simulink model "afe_abc_inv_pmsm"  (R2024b)
settings: Solver=ode1be  StartTime=0.0  StopTime=simlength  FixedStep=tc  MaxStep=tc
undefined symbols (not defined in the file): Adrso, Amplitude_U, Amplitude_V, Amplitude_W, Aresd, b, Bresd, Cresd, Crso, CTRPIFF_CLIP_RELEASE, dead_time_AFE, dead_time_INV, deepNEGeta, deepNEGxi, deepPOSxi, emf_fb_p, emf_fb_p_ccaller_1, emf_fb_p_ccaller_2, emf_p, emf_p_ccaller_1, emf_p_ccaller_2, end_time_LVRT, fPWM_AFE, fPWM_INV, g0_161Hz, g0_500Hz, g1_161Hz, g1_500Hz, i_grid_neg_eta_lim, i_grid_neg_eta_red_lim, i_grid_neg_xi_lim, i_grid_neg_xi_red_lim, i_grid_pos_eta_lim, i_grid_pos_eta_red_lim, ibez, id_lim, ieta_neg_ref_lim, ieta_pos_ref_lim, Igrid_phase_normalization_factor, iq_lim, ixi_pos_ref_lim, Jm, k_frt_ref, kg, ki_afe, ki_i, ki_rc_neg_grid, ki_rc_pos_grid, ki_vs, ki_w, kp_afe, kp_i, kp_rc_neg_grid, kp_rc_pos_grid, kp_vs, kp_w, kw, l1, l2, Ld_norm ... (+45)
libraries: fl_lib x115, nesl_utility x75, cstblocks x14, simulink x13, single_phase_transformer_lib x3, threephase_inductor_lib x2, flexshaft_lib x1, pmsm_uvw_with_harmonics_lib x1
(part 8 of 10)

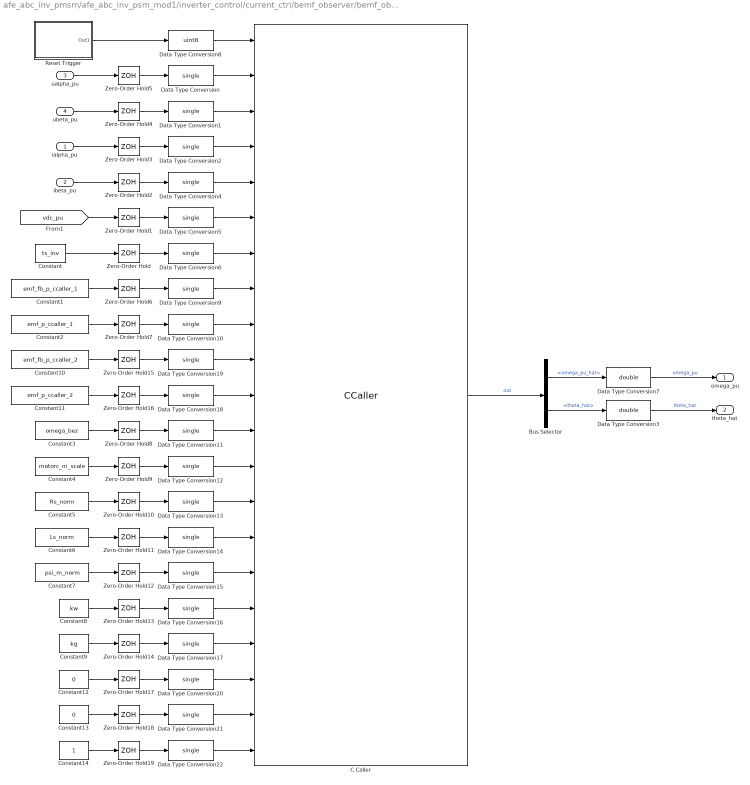
== system afe_abc_inv_pmsm/afe_abc_inv_psm_mod1/inverter_control/current_ctrl/bemf_observer/bemf_observer_ccaller ==
  ialpha_pu : Inport
  ibeta_pu : Inport  Port=2
  ualpha_pu : Inport  Port=3
  ubeta_pu : Inport  Port=4
  Bus Selector : BusSelector  OutputSignals=omega_pu_hat,theta_hat
  C Caller : CCaller  FunctionName=bemf_obsv_process_simulink  PortSpecificationStruct="%)30     .    N\"8   8    (     @         %    \"    !8    !     0         %  0 \"0    $    _    07)G3F%M90  4&]R=$YA;64 4V-O<&4     26YD97@     5'EP90      4VEZ90      27-';&]B86P   X    P    !@    @    $          4    (     0    ,    !         !   P!O=70 #@   #     &    \"     0         !0    @    !     P    $         $  # &]U=  .    .     8    (    !          %    \"     $    &     0         0  ...(+12985 chars)"  SampleTime=ts_inv
  Constant : Constant  Value=ts_inv
  Constant1 : Constant  Value=emf_fb_p_ccaller_1
  Constant10 : Constant  Value=emf_fb_p_ccaller_2
  Constant11 : Constant  Value=emf_p_ccaller_2
  Constant12 : Constant  Value=0
  Constant13 : Constant  Value=0
  Constant14 : Constant
  Constant2 : Constant  Value=emf_p_ccaller_1
  Constant3 : Constant  Value=omega_bez
  Constant4 : Constant  Value=motorc_m_scale
  Constant5 : Constant  Value=Rs_norm
  Constant6 : Constant  Value=Ls_norm
  Constant7 : Constant  Value=psi_m_norm
  Constant8 : Constant  Value=kw
  Constant9 : Constant  Value=kg
  Data Type Conversion{,1..2,4..6,9..22} (20 alike) : DataTypeConversion  OutDataTypeStr=single  SaturateOnIntegerOverflow=off  RndMeth=Floor
  Data Type Conversion3 : DataTypeConversion  OutDataTypeStr=double  SaturateOnIntegerOverflow=off  RndMeth=Floor
  Data Type Conversion7 : DataTypeConversion  OutDataTypeStr=double  SaturateOnIntegerOverflow=off  RndMeth=Floor
  Data Type Conversion8 : DataTypeConversion  OutDataTypeStr=uint8  SaturateOnIntegerOverflow=off  RndMeth=Floor
  Reset Trigger : Subsystem
  Zero-Order Hold{,1..19} (20 alike) : ZeroOrderHold  SampleTime=ts_inv
  omega_pu : Outport
  theta_hat : Outport  Port=2
  wires:
  Data Type Conversion5/1 -> C Caller/6
  Data Type Conversion/1 -> C Caller/2
  C Caller/1 -> Bus Selector/1  "out"
  Data Type Conversion1/1 -> C Caller/3
  Data Type Conversion4/1 -> C Caller/5
  Data Type Conversion2/1 -> C Caller/4
  Data Type Conversion6/1 -> C Caller/7
  Zero-Order Hold/1 -> Data Type Conversion6/1
  Zero-Order Hold5/1 -> Data Type Conversion/1
  Zero-Order Hold4/1 -> Data Type Conversion1/1
  Zero-Order Hold3/1 -> Data Type Conversion2/1
  Zero-Order Hold2/1 -> Data Type Conversion4/1
  Zero-Order Hold1/1 -> Data Type Conversion5/1
  [vdc_pu] -> Zero-Order Hold1/1
  Constant/1 -> Zero-Order Hold/1
  ualpha_pu/1 -> Zero-Order Hold5/1
  ialpha_pu/1 -> Zero-Order Hold3/1
  ubeta_pu/1 -> Zero-Order Hold4/1
  ibeta_pu/1 -> Zero-Order Hold2/1
  Bus Selector/2 -> Data Type Conversion3/1  "<theta_hat>"
  Bus Selector/1 -> Data Type Conversion7/1  "<omega_pu_hat>"
  Data Type Conversion7/1 -> omega_pu/1  "omega_pu"
  Data Type Conversion3/1 -> theta_hat/1  "theta_hat"
  Reset Trigger/1(Out1) -> Data Type Conversion8/1
  Data Type Conversion8/1 -> C Caller/1
  Constant1/1 -> Zero-Order Hold6/1
  Zero-Order Hold6/1 -> Data Type Conversion9/1
  Data Type Conversion9/1 -> C Caller/8
  Data Type Conversion10/1 -> C Caller/9
  Zero-Order Hold7/1 -> Data Type Conversion10/1
  Zero-Order Hold8/1 -> Data Type Conversion11/1
  Zero-Order Hold9/1 -> Data Type Conversion12/1
  Zero-Order Hold10/1 -> Data Type Conversion13/1
  Zero-Order Hold11/1 -> Data Type Conversion14/1
  Zero-Order Hold12/1 -> Data Type Conversion15/1
  Zero-Order Hold13/1 -> Data Type Conversion16/1
  Zero-Order Hold14/1 -> Data Type Conversion17/1
  Constant2/1 -> Zero-Order Hold7/1
  Constant3/1 -> Zero-Order Hold8/1
  Constant4/1 -> Zero-Order Hold9/1
  Constant5/1 -> Zero-Order Hold10/1
  Constant6/1 -> Zero-Order Hold11/1
  Constant7/1 -> Zero-Order Hold12/1
  Constant8/1 -> Zero-Order Hold13/1
  Constant9/1 -> Zero-Order Hold14/1
  Constant11/1 -> Zero-Order Hold16/1
  Zero-Order Hold16/1 -> Data Type Conversion18/1
  Zero-Order Hold15/1 -> Data Type Conversion19/1
  Constant10/1 -> Zero-Order Hold15/1
  Data Type Conversion19/1 -> C Caller/10
  Data Type Conversion18/1 -> C Caller/11
  Data Type Conversion11/1 -> C Caller/12
  Data Type Conversion12/1 -> C Caller/13
  Data Type Conversion13/1 -> C Caller/14
  Data Type Conversion14/1 -> C Caller/15
  Data Type Conversion15/1 -> C Caller/16
  Data Type Conversion16/1 -> C Caller/17
  Data Type Conversion17/1 -> C Caller/18
  Data Type Conversion20/1 -> C Caller/19
  Constant12/1 -> Zero-Order Hold17/1
  Zero-Order Hold17/1 -> Data Type Conversion20/1
  Zero-Order Hold18/1 -> Data Type Conversion21/1
  Constant13/1 -> Zero-Order Hold18/1
  Data Type Conversion21/1 -> C Caller/20
  Constant14/1 -> Zero-Order Hold19/1
  Zero-Order Hold19/1 -> Data Type Conversion22/1
  Data Type Conversion22/1 -> C Caller/21

== system afe_abc_inv_pmsm/afe_abc_inv_psm_mod1/inverter_control/current_ctrl/bemf_observer/double_integrator_observer ==
  theta : Inport
  Dead Zone : DeadZone  LowerValue=-0.01  UpperValue=0.01
  Gain : Gain  Gain=kw
  Gain1 : Gain  Gain=kg
  Gain2 : Gain  Gain=omega_bez
  Gain3 : Gain  Gain=1/omega_bez
  Gain5 : Gain  Gain=ts_inv
  Sum : Sum  Inputs=-+|
  Sum1 : Sum  Inputs=|++
  Sum2 : Sum  Inputs=|++
  Sum8 : Sum  Inputs=++|
  Unit Delay1 : UnitDelay  InitialCondition=pi  SampleTime=ts_inv  HasFrameUpgradeWarning=on
  Unit Delay2 : UnitDelay  SampleTime=ts_inv  HasFrameUpgradeWarning=on
  bounder1 : MATLAB Function  TreatAsAtomicUnit=on  SystemSampleTime=ts_inv
  bounder2 : MATLAB Function  TreatAsAtomicUnit=on  SystemSampleTime=ts_inv
  omega_pu_hat : Outport  VectorParamsAs1DForOutWhenUnconnected=off
  theta_hat : Outport  Port=2  VectorParamsAs1DForOutWhenUnconnected=off
  wires:
  Gain1/1 -> Sum2/1
  theta/1 -> Sum/2  "theta_bemf"
  Sum8/1 -> Unit Delay1/1
  Unit Delay1/1 -> bounder2/1(u)
  Sum1/1 -> Unit Delay2/1
  Gain/1 -> Gain3/1
  Unit Delay2/1 -> omega_pu_hat/1, Sum1/2, Gain5/1
  Sum2/1 -> Sum8/2
  bounder2/1(y) -> Sum2/2, theta_hat/1, Sum/1  "theta_hat"
  bounder1/1(y) -> Gain1/1, Gain/1
  Gain2/1 -> Sum8/1
  Gain3/1 -> Sum1/1
  Gain5/1 -> Gain2/1
  Sum/1 -> bounder1/1(u)

== system afe_abc_inv_pmsm/afe_abc_inv_psm_mod1/inverter_control/current_ctrl/bemf_observer/phase_fault ==
  theta_pmsm : Inport
  Manual Switch : ManualSwitch
  Manual Switch1 : ManualSwitch  CurrentSetting=0
  drop_phase_zerofor_delta_time : Subsystem
  hold_phase_for_delta_time : Subsystem
  loss_phase : Subsystem
  theta : Outport
  wires:
  theta_pmsm/1 -> drop_phase_zerofor_delta_time/1(theta_pmsm), loss_phase/1(theta_pmsm), hold_phase_for_delta_time/1(theta_pmsm)
  drop_phase_zerofor_delta_time/1(theta) -> Manual Switch/1
  hold_phase_for_delta_time/1(theta) -> Manual Switch/2
  Manual Switch/1 -> Manual Switch1/1
  loss_phase/1(theta) -> Manual Switch1/2
  Manual Switch1/1 -> theta/1

== system afe_abc_inv_pmsm/afe_abc_inv_psm_mod1/inverter_control/current_ctrl/current_ctrl/MTPA ==
  iq_ref : Inport
  Gain1 : Gain  Gain=1/(Ld_norm - Lq_norm)/2
  Gain2 : Gain  Gain=1/(Ld_norm - Lq_norm)/2
  Gain3 : Gain  Gain=-1
  Math Function1 : Math  Operator=magnitude^2  SignedPower=on
  Math Function4 : Math  Operator=magnitude^2  SignedPower=on
  Sqrt : Sqrt
  Sum : Sum  Inputs=|++
  Sum1 : Sum  Inputs=|-+
  id_ref_pu < x < 0 : Saturate  UpperLimit=0  LowerLimit=-id_lim
  Id_ref_mtpa : Outport  VectorParamsAs1DForOutWhenUnconnected=off
  wires:
  Sum1/1 -> Gain3/1
  id_ref_pu < x < 0/1 -> Id_ref_mtpa/1
  Math Function4/1 -> Sum/1
  Math Function1/1 -> Sum/2
  Gain1/1 -> Math Function4/1
  Sum/1 -> Sqrt/1
  Sqrt/1 -> Sum1/2
  iq_ref/1 -> Math Function1/1
  Gain2/1 -> Sum1/1
  [omega_hat_pu] -> Gain1/1, Gain2/1
  Gain3/1 -> id_ref_pu < x < 0/1

== system afe_abc_inv_pmsm/afe_abc_inv_psm_mod1/inverter_control/current_ctrl/current_ctrl/dq_pi_with_vector_antiwindup ==
  id_ref : Inport
  id : Inport  Port=2
  iq_ref : Inport  Port=3
  iq : Inport  Port=4
  Variant Source : VariantSource
  Variant Source1 : VariantSource
  dq_vector_pi : Subsystem
  dq_vector_pi_ccaller : Subsystem
  simulink/Ccaller VectorPI : Scope  NumInputPorts=2
  ctrl_d_u : Outport
  ctrl_q_u : Outport  Port=2
  wires:
  id/1 -> dq_vector_pi_ccaller/1(id), dq_vector_pi/1(id)  "id"
  id_ref/1 -> dq_vector_pi_ccaller/2(id_ref), dq_vector_pi/2(id_ref)  "id_ref"
  iq/1 -> dq_vector_pi_ccaller/3(iq), dq_vector_pi/3(iq)  "iq"
  iq_ref/1 -> dq_vector_pi/4(iq_ref), dq_vector_pi_ccaller/4(iq_ref)  "iq_ref"
  dq_vector_pi/1(md_sat) -> Variant Source/1
  dq_vector_pi_ccaller/2(uq_ctrl_out) -> Variant Source1/2
  dq_vector_pi/2(mq_sat) -> Variant Source1/1
  dq_vector_pi_ccaller/1(ud_ctrl_out) -> Variant Source/2
  Variant Source/1 -> ctrl_d_u/1, simulink/Ccaller VectorPI/1
  Variant Source1/1 -> simulink/Ccaller VectorPI/2, ctrl_q_u/1

== system afe_abc_inv_pmsm/afe_abc_inv_psm_mod1/inverter_control/current_ctrl/current_ctrl/id_ref ==
  id_mtpa : Inport
  Constant : Constant  Value=0
  Variant Source : VariantSource
  id_ref : Outport
  wires:
  Variant Source/1 -> id_ref/1
  id_mtpa/1 -> Variant Source/1
  Constant/1 -> Variant Source/2

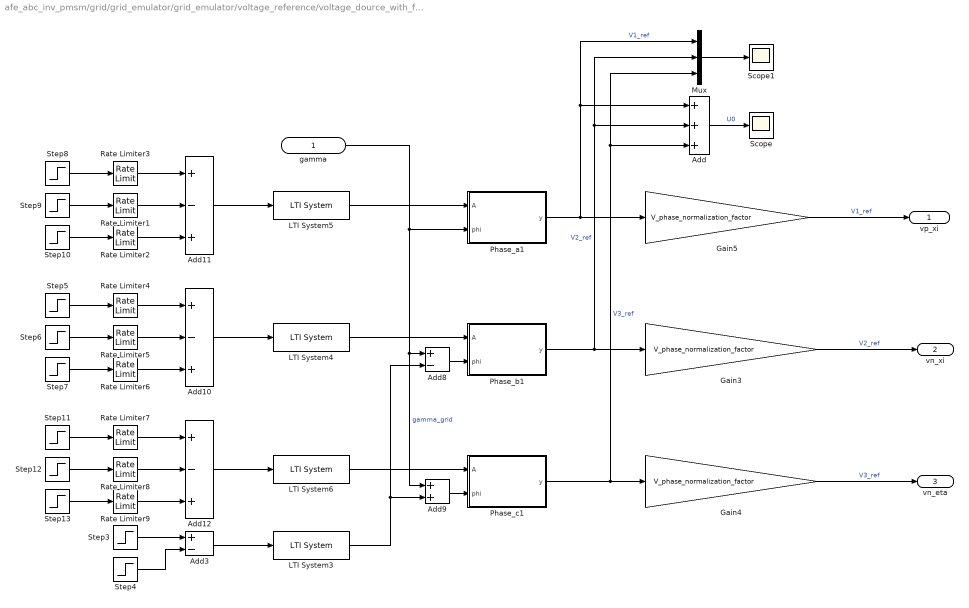
== system afe_abc_inv_pmsm/grid/grid_emulator/grid_emulator/voltage_reference/voltage_dource_with_frt ==
  gamma : Inport
  Add : Sum  Inputs=+++
  Add10 : Sum  Inputs=+-+
  Add11 : Sum  Inputs=+-+
  Add12 : Sum  Inputs=+-+
  Add3 : Sum  Inputs=+-
  Add8 : Sum  Inputs=+-
  Add9 : Sum
  Gain3 : Gain  Gain=V_phase_normalization_factor
  Gain4 : Gain  Gain=V_phase_normalization_factor
  Gain5 : Gain  Gain=V_phase_normalization_factor
  LTI System{3..6} (4 alike) : cstblocks/LTI System  sys=LVRT_flt_ss_c  IC=[0]  PadeOrder=0
  Mux : Mux  Inputs=3
  Phase_a1 : MATLAB Function  TreatAsAtomicUnit=on
  Phase_b1 : MATLAB Function  TreatAsAtomicUnit=on
  Phase_c1 : MATLAB Function  TreatAsAtomicUnit=on
  Rate Limiter{1..9} (9 alike) : RateLimiter  RisingSlewLimit=Vemu_ref_norm/t_ramp  FallingSlewLimit=-Vemu_ref_norm/t_ramp  SampleTimeMode=inherited
  Scope : Scope
  Scope1 : Scope
  Step10 : Step  Time=end_time_LVRT  After=Vemu_ref_norm*(1-Amplitude_U)  SampleTime=0
  Step11 : Step  Time=0  After=Vemu_ref_norm  SampleTime=0
  Step12 : Step  Time=start_time_LVRT  After=Vemu_ref_norm*(1-Amplitude_W)  SampleTime=0
  Step13 : Step  Time=end_time_LVRT  After=Vemu_ref_norm*(1-Amplitude_W)  SampleTime=0
  Step3 : Step  Time=start_time_LVRT  After=Phase_shift  SampleTime=0
  Step4 : Step  Time=end_time_LVRT  After=Phase_shift  SampleTime=0
  Step5 : Step  Time=0  After=Vemu_ref_norm  SampleTime=0
  Step6 : Step  Time=start_time_LVRT  After=Vemu_ref_norm*(1-Amplitude_V)  SampleTime=0
  Step7 : Step  Time=end_time_LVRT  After=Vemu_ref_norm*(1-Amplitude_V)  SampleTime=0
  Step8 : Step  Time=0  After=Vemu_ref_norm  SampleTime=0
  Step9 : Step  Time=start_time_LVRT  After=Vemu_ref_norm*(1-Amplitude_U)  SampleTime=0
  vp_xi : Outport  VectorParamsAs1DForOutWhenUnconnected=off
  vn_xi : Outport  Port=2  VectorParamsAs1DForOutWhenUnconnected=off
  vn_eta : Outport  Port=3  VectorParamsAs1DForOutWhenUnconnected=off
  wires:
  Phase_c1/1(y) -> Mux/3, Add/3, Gain4/1  "V3_ref"
  LTI System6/1 -> Phase_c1/1(A)
  gamma/1 -> Add9/1, Add8/1, Phase_a1/2(phi)  "gamma_grid"
  Add9/1 -> Phase_c1/2(phi)
  Add8/1 -> Phase_b1/2(phi)
  Phase_b1/1(y) -> Mux/2, Add/2, Gain3/1  "V2_ref"
  Phase_a1/1(y) -> Mux/1, Add/1, Gain5/1  "V1_ref"
  LTI System4/1 -> Phase_b1/1(A)
  Step5/1 -> Rate Limiter4/1
  Step6/1 -> Rate Limiter5/1
  Step7/1 -> Rate Limiter6/1
  Add10/1 -> LTI System4/1
  Step8/1 -> Rate Limiter3/1
  Add11/1 -> LTI System5/1
  Step9/1 -> Rate Limiter1/1
  Step10/1 -> Rate Limiter2/1
  LTI System5/1 -> Phase_a1/1(A)
  Add12/1 -> LTI System6/1
  Rate Limiter3/1 -> Add11/1
  Rate Limiter1/1 -> Add11/2
  Rate Limiter2/1 -> Add11/3
  Rate Limiter4/1 -> Add10/1
  Rate Limiter5/1 -> Add10/2
  Rate Limiter6/1 -> Add10/3
  Step12/1 -> Rate Limiter8/1
  Rate Limiter8/1 -> Add12/2
  Step13/1 -> Rate Limiter9/1
  Rate Limiter9/1 -> Add12/3
  Step11/1 -> Rate Limiter7/1
  Rate Limiter7/1 -> Add12/1
  Gain5/1 -> vp_xi/1  "V1_ref"
  Gain3/1 -> vn_xi/1  "V2_ref"
  Gain4/1 -> vn_eta/1  "V3_ref"
  Add3/1 -> LTI System3/1
  Step3/1 -> Add3/1
  Step4/1 -> Add3/2
  LTI System3/1 -> Add9/2, Add8/2
  Add/1 -> Scope/1  "U0"
  Mux/1 -> Scope1/1

== system afe_abc_inv_pmsm/afe_abc_inv_psm_mod1/afe_control/current_sequence_avg/average_filter_ccaller/Moving Average Filter5/Enabled Subsystem ==
  In1 : Inport
  Enable : EnablePort
  Constant2 : Constant
  Divide : Product  Inputs=*/
  Gain1 : Gain  Gain=1/(2*pi)
  Gain9 : Gain  Gain=mavarage_filter_frequency_base_order
  Zero-Order Hold : ZeroOrderHold  SampleTime=ts_afe
  Out1 : Outport
  wires:
  Gain1/1 -> Gain9/1
  Zero-Order Hold/1 -> Out1/1  "period"
  Gain9/1 -> Divide/2
  In1/1 -> Gain1/1  "Omega_el"
  Divide/1 -> Zero-Order Hold/1
  Constant2/1 -> Divide/1

== system afe_abc_inv_pmsm/afe_abc_inv_psm_mod1/afe_control/current_sequence_avg/average_filter_ccaller/Moving Average Filter5/Reset Trigger ==
  Clock : Clock
  Constant1 : Constant  Value=simlength
  Constant3 : Constant  Value=0
  Constant4 : Constant
  Mod : Math  Operator=mod
  Switch : Switch  Criteria=u2 ~= 0  SaturateOnIntegerOverflow=off  InputSameDT=off
  Zero-Order Hold : ZeroOrderHold  SampleTime=ts_afe
  Out1 : Outport
  wires:
  Constant1/1 -> Mod/2
  Switch/1 -> Out1/1  "Reset"
  Clock/1 -> Zero-Order Hold/1
  Mod/1 -> Switch/2
  Constant4/1 -> Switch/3
  Zero-Order Hold/1 -> Mod/1
  Constant3/1 -> Switch/1

== system afe_abc_inv_pmsm/afe_abc_inv_psm_mod1/afe_control/current_sequence_avg/average_filter_ccaller/Moving Average Filter6/Enabled Subsystem ==
  In1 : Inport
  Enable : EnablePort
  Constant2 : Constant
  Divide : Product  Inputs=*/
  Gain1 : Gain  Gain=1/(2*pi)
  Gain9 : Gain  Gain=mavarage_filter_frequency_base_order
  Zero-Order Hold : ZeroOrderHold  SampleTime=ts_afe
  Out1 : Outport
  wires:
  Constant2/1 -> Divide/1
  Divide/1 -> Zero-Order Hold/1
  In1/1 -> Gain1/1  "Omega_el"
  Gain9/1 -> Divide/2
  Zero-Order Hold/1 -> Out1/1  "period"
  Gain1/1 -> Gain9/1

== system afe_abc_inv_pmsm/afe_abc_inv_psm_mod1/afe_control/current_sequence_avg/average_filter_ccaller/Moving Average Filter6/Reset Trigger ==
  Clock : Clock
  Constant1 : Constant  Value=simlength
  Constant3 : Constant  Value=0
  Constant4 : Constant
  Mod : Math  Operator=mod
  Switch : Switch  Criteria=u2 ~= 0  SaturateOnIntegerOverflow=off  InputSameDT=off
  Zero-Order Hold : ZeroOrderHold  SampleTime=ts_afe
  Out1 : Outport
  wires:
  Constant3/1 -> Switch/1
  Zero-Order Hold/1 -> Mod/1
  Constant4/1 -> Switch/3
  Mod/1 -> Switch/2
  Clock/1 -> Zero-Order Hold/1
  Switch/1 -> Out1/1  "Reset"
  Constant1/1 -> Mod/2

== system afe_abc_inv_pmsm/afe_abc_inv_psm_mod1/afe_control/current_sequence_avg/average_filter_ccaller/Moving Average Filter7/Enabled Subsystem ==
  In1 : Inport
  Enable : EnablePort
  Constant2 : Constant
  Divide : Product  Inputs=*/
  Gain1 : Gain  Gain=1/(2*pi)
  Gain9 : Gain  Gain=mavarage_filter_frequency_base_order
  Zero-Order Hold : ZeroOrderHold  SampleTime=ts_afe
  Out1 : Outport
  wires:
  Gain1/1 -> Gain9/1
  Zero-Order Hold/1 -> Out1/1  "period"
  Gain9/1 -> Divide/2
  In1/1 -> Gain1/1  "Omega_el"
  Divide/1 -> Zero-Order Hold/1
  Constant2/1 -> Divide/1

== system afe_abc_inv_pmsm/afe_abc_inv_psm_mod1/afe_control/current_sequence_avg/average_filter_ccaller/Moving Average Filter7/Reset Trigger ==
  Clock : Clock
  Constant1 : Constant  Value=simlength
  Constant3 : Constant  Value=0
  Constant4 : Constant
  Mod : Math  Operator=mod
  Switch : Switch  Criteria=u2 ~= 0  SaturateOnIntegerOverflow=off  InputSameDT=off
  Zero-Order Hold : ZeroOrderHold  SampleTime=ts_afe
  Out1 : Outport
  wires:
  Constant1/1 -> Mod/2
  Switch/1 -> Out1/1  "Reset"
  Clock/1 -> Zero-Order Hold/1
  Mod/1 -> Switch/2
  Constant4/1 -> Switch/3
  Zero-Order Hold/1 -> Mod/1
  Constant3/1 -> Switch/1

== system afe_abc_inv_pmsm/afe_abc_inv_psm_mod1/afe_control/current_sequence_avg/average_filter_ccaller/Moving Average Filter8/Enabled Subsystem ==
  In1 : Inport
  Enable : EnablePort
  Constant2 : Constant
  Divide : Product  Inputs=*/
  Gain1 : Gain  Gain=1/(2*pi)
  Gain9 : Gain  Gain=mavarage_filter_frequency_base_order
  Zero-Order Hold : ZeroOrderHold  SampleTime=ts_afe
  Out1 : Outport
  wires:
  Constant2/1 -> Divide/1
  Divide/1 -> Zero-Order Hold/1
  In1/1 -> Gain1/1  "Omega_el"
  Gain9/1 -> Divide/2
  Zero-Order Hold/1 -> Out1/1  "period"
  Gain1/1 -> Gain9/1

== system afe_abc_inv_pmsm/afe_abc_inv_psm_mod1/afe_control/current_sequence_avg/average_filter_ccaller/Moving Average Filter8/Reset Trigger ==
  Clock : Clock
  Constant1 : Constant  Value=simlength
  Constant3 : Constant  Value=0
  Constant4 : Constant
  Mod : Math  Operator=mod
  Switch : Switch  Criteria=u2 ~= 0  SaturateOnIntegerOverflow=off  InputSameDT=off
  Zero-Order Hold : ZeroOrderHold  SampleTime=ts_afe
  Out1 : Outport
  wires:
  Constant3/1 -> Switch/1
  Zero-Order Hold/1 -> Mod/1
  Constant4/1 -> Switch/3
  Mod/1 -> Switch/2
  Clock/1 -> Zero-Order Hold/1
  Switch/1 -> Out1/1  "Reset"
  Constant1/1 -> Mod/2

== system afe_abc_inv_pmsm/afe_abc_inv_psm_mod1/afe_control/grid_voltage_phase_lock_loops/DDSRF-PLL/pll_stageA/mormalization_and_transformation ==
  ug_a : Inport
  ug_b : Inport  Port=2
  ug_c : Inport  Port=3
  Gain1 : Gain  Gain=1/Vgrid_phase_normalization_factor
  Gain2 : Gain  Gain=1/Vgrid_phase_normalization_factor
  Gain3 : Gain  Gain=1/Vgrid_phase_normalization_factor
  Zero-Order Hold : ZeroOrderHold  SampleTime=ts_afe
  Zero-Order Hold1 : ZeroOrderHold  SampleTime=ts_afe
  Zero-Order Hold2 : ZeroOrderHold  SampleTime=ts_afe
  abc2alphabeta : MATLAB Function  TreatAsAtomicUnit=on
  ug_alpha : Outport  VectorParamsAs1DForOutWhenUnconnected=off
  ug_beta : Outport  Port=2  VectorParamsAs1DForOutWhenUnconnected=off
  wires:
  abc2alphabeta/1(alpha) -> ug_alpha/1  "u_grid_alpha"
  abc2alphabeta/2(beta) -> ug_beta/1  "u_grid_beta"
  Gain3/1 -> abc2alphabeta/3(c)
  Gain2/1 -> abc2alphabeta/2(b)
  Gain1/1 -> abc2alphabeta/1(a)
  Zero-Order Hold2/1 -> Gain3/1
  Zero-Order Hold1/1 -> Gain2/1
  Zero-Order Hold/1 -> Gain1/1
  ug_b/1 -> Zero-Order Hold1/1
  ug_c/1 -> Zero-Order Hold2/1
  ug_a/1 -> Zero-Order Hold/1

== system afe_abc_inv_pmsm/afe_abc_inv_psm_mod1/afe_control/grid_voltage_phase_lock_loops/DDSRF-PLL/pll_stageA/sequences ==
  u_grid_alpha : Inport
  u_grid_beta : Inport  Port=2
  phase_angle : Inport  Port=3
  ddsrf : Subsystem
  u_grid_pos_xi : Outport
  u_grid_pos_eta : Outport  Port=2
  wires:
  phase_angle/1 -> ddsrf/3(phase_angle)  "phase_angle"
  u_grid_beta/1 -> ddsrf/2(u_grid_beta)  "u_grid_beta"
  u_grid_alpha/1 -> ddsrf/1(u_grid_alpha)  "u_grid_alpha"
  ddsrf/2(u_grid_pos_eta) -> u_grid_pos_eta/1  "u_grid_pos_eta"
  ddsrf/1(u_grid_pos_xi) -> u_grid_pos_xi/1  "u_grid_pos_xi"

== system afe_abc_inv_pmsm/afe_abc_inv_psm_mod1/afe_control/grid_voltage_phase_lock_loops/DDSRF-PLL/pll_stageB/double_integrator_observer ==
  theta : Inport
  Gain : Gain  Gain=Ldrso  Multiplication=Matrix(K*u)
  Gain1 : Gain  Gain=Adrso  Multiplication=Matrix(K*u)
  Gain2 : Gain  Gain=Crso  Multiplication=Matrix(K*u)
  Selector : Selector  InputPortWidth=2  IndexOptions=Index vector (dialog)  Indices=2  OutputSizes=1
  Sum : Sum  Inputs=-+|
  Sum1 : Sum  Inputs=|++
  Unit Delay : UnitDelay  SampleTime=ts_afe  HasFrameUpgradeWarning=on
  Zero-Order Hold : ZeroOrderHold  SampleTime=ts_afe
  bounder1 : MATLAB Function  TreatAsAtomicUnit=on  SystemSampleTime=ts_afe
  bounder2 : MATLAB Function  TreatAsAtomicUnit=on  SystemSampleTime=ts_afe
  omega_hat : Outport
  wires:
  bounder2/1(y) -> Sum/1  "theta_hat_bounded"
  bounder1/1(y) -> Gain/1  "e_bounded"
  Zero-Order Hold/1 -> Sum/2  "theta_dsp"
  theta/1 -> Zero-Order Hold/1  "theta"
  Unit Delay/1 -> Gain2/1, Selector/1, Gain1/1
  Sum/1 -> bounder1/1(u)  "e"
  Sum1/1 -> Unit Delay/1
  Gain1/1 -> Sum1/2
  Gain2/1 -> bounder2/1(u)  "theta_hat"
  Selector/1 -> omega_hat/1
  Gain/1 -> Sum1/1

== system afe_abc_inv_pmsm/afe_abc_inv_psm_mod1/afe_control/grid_voltage_phase_lock_loops/DQ-PLL/pll_stageA/mormalization_and_transformation ==
  ug_a : Inport
  ug_b : Inport  Port=2
  ug_c : Inport  Port=3
  Gain1 : Gain  Gain=1/Vgrid_phase_normalization_factor
  Gain2 : Gain  Gain=1/Vgrid_phase_normalization_factor
  Gain3 : Gain  Gain=1/Vgrid_phase_normalization_factor
  Mux : Mux  Inputs=3
  Zero-Order Hold : ZeroOrderHold  SampleTime=ts_afe
  Zero-Order Hold1 : ZeroOrderHold  SampleTime=ts_afe
  Zero-Order Hold2 : ZeroOrderHold  SampleTime=ts_afe
  abc2alphabeta : MATLAB Function  TreatAsAtomicUnit=on  SystemSampleTime=ts_afe
  u_500Hz_flt : Subsystem
  u_500Hz_flt1 : Subsystem
  u_500Hz_flt2 : Subsystem
  ug_alpha : Outport  VectorParamsAs1DForOutWhenUnconnected=off
  ug_beta : Outport  Port=2  VectorParamsAs1DForOutWhenUnconnected=off
  tag scope: v_grid_ff_abc=global
  wires:
  ug_a/1 -> Zero-Order Hold/1
  ug_c/1 -> Zero-Order Hold2/1
  ug_b/1 -> Zero-Order Hold1/1
  Zero-Order Hold/1 -> Gain1/1
  Zero-Order Hold1/1 -> Gain2/1
  Zero-Order Hold2/1 -> Gain3/1
  abc2alphabeta/2(beta) -> ug_beta/1  "u_grid_beta"
  abc2alphabeta/1(alpha) -> ug_alpha/1  "u_grid_alpha"
  u_500Hz_flt1/1(output) -> Mux/2
  u_500Hz_flt2/1(output) -> Mux/3
  u_500Hz_flt/1(output) -> Mux/1
  Gain3/1 -> u_500Hz_flt2/1(input), abc2alphabeta/3(c)
  Gain2/1 -> u_500Hz_flt1/1(input), abc2alphabeta/2(b)
  Mux/1 -> [v_grid_ff_abc]
  Gain1/1 -> u_500Hz_flt/1(input), abc2alphabeta/1(a)

== system afe_abc_inv_pmsm/afe_abc_inv_psm_mod1/afe_control/grid_voltage_phase_lock_loops/DQ-PLL/pll_stageA/sequences ==
  u_grid_alpha : Inport
  u_grid_beta : Inport  Port=2
  gamma_grid : Inport  Port=3
  alphabeta2xieta : Subsystem
  u_grid_pos_xi : Outport
  u_grid_pos_eta : Outport  Port=2
  wires:
  alphabeta2xieta/1(xi) -> u_grid_pos_xi/1  "u_grid_pos_xi"
  alphabeta2xieta/2(eta) -> u_grid_pos_eta/1  "u_grid_pos_eta"
  u_grid_alpha/1 -> alphabeta2xieta/1(alpha)  "u_grid_alpha"
  u_grid_beta/1 -> alphabeta2xieta/2(beta)  "u_grid_beta"
  gamma_grid/1 -> alphabeta2xieta/3(gamma)  "gamma_grid"

== system afe_abc_inv_pmsm/afe_abc_inv_psm_mod1/afe_control/grid_voltage_phase_lock_loops/DQ-PLL/pll_stageB/double_integrator_observer ==
  theta : Inport
  Gain : Gain  Gain=Ldrso  Multiplication=Matrix(K*u)
  Gain1 : Gain  Gain=Adrso  Multiplication=Matrix(K*u)
  Gain2 : Gain  Gain=Crso  Multiplication=Matrix(K*u)
  Selector : Selector  InputPortWidth=2  IndexOptions=Index vector (dialog)  Indices=2  OutputSizes=1
  Sum : Sum  Inputs=-+|
  Sum1 : Sum  Inputs=|++
  Unit Delay : UnitDelay  SampleTime=ts_afe  HasFrameUpgradeWarning=on
  Zero-Order Hold : ZeroOrderHold  SampleTime=ts_afe
  bounder1 : MATLAB Function  TreatAsAtomicUnit=on  SystemSampleTime=ts_afe
  bounder2 : MATLAB Function  TreatAsAtomicUnit=on  SystemSampleTime=ts_afe
  omega_hat : Outport
  wires:
  Gain/1 -> Sum1/1
  Selector/1 -> omega_hat/1
  Gain2/1 -> bounder2/1(u)  "theta_hat"
  Gain1/1 -> Sum1/2
  Sum1/1 -> Unit Delay/1
  Sum/1 -> bounder1/1(u)  "e"
  Unit Delay/1 -> Gain1/1, Selector/1, Gain2/1
  theta/1 -> Zero-Order Hold/1  "theta"
  Zero-Order Hold/1 -> Sum/2  "theta_dsp"
  bounder1/1(y) -> Gain/1  "e_bounded"
  bounder2/1(y) -> Sum/1  "theta_hat_bounded"

== system afe_abc_inv_pmsm/afe_abc_inv_psm_mod1/afe_control/voltage_sequence_avg/average_filter_ccaller/Moving Average Filter1/Enabled Subsystem ==
  In1 : Inport
  Enable : EnablePort
  Constant2 : Constant
  Divide : Product  Inputs=*/
  Gain1 : Gain  Gain=1/(2*pi)
  Gain9 : Gain  Gain=mavarage_filter_frequency_base_order
  Zero-Order Hold : ZeroOrderHold  SampleTime=ts_afe
  Out1 : Outport
  wires:
  Gain1/1 -> Gain9/1
  Zero-Order Hold/1 -> Out1/1  "period"
  Gain9/1 -> Divide/2
  In1/1 -> Gain1/1  "Omega_el"
  Divide/1 -> Zero-Order Hold/1
  Constant2/1 -> Divide/1

== system afe_abc_inv_pmsm/afe_abc_inv_psm_mod1/afe_control/voltage_sequence_avg/average_filter_ccaller/Moving Average Filter1/Reset Trigger ==
  Clock : Clock
  Constant1 : Constant  Value=simlength
  Constant3 : Constant  Value=0
  Constant4 : Constant
  Mod : Math  Operator=mod
  Switch : Switch  Criteria=u2 ~= 0  SaturateOnIntegerOverflow=off  InputSameDT=off
  Zero-Order Hold : ZeroOrderHold  SampleTime=ts_afe
  Out1 : Outport
  wires:
  Constant1/1 -> Mod/2
  Switch/1 -> Out1/1  "Reset"
  Clock/1 -> Zero-Order Hold/1
  Mod/1 -> Switch/2
  Constant4/1 -> Switch/3
  Zero-Order Hold/1 -> Mod/1
  Constant3/1 -> Switch/1

== system afe_abc_inv_pmsm/afe_abc_inv_psm_mod1/afe_control/voltage_sequence_avg/average_filter_ccaller/Moving Average Filter2/Enabled Subsystem ==
  In1 : Inport
  Enable : EnablePort
  Constant2 : Constant
  Divide : Product  Inputs=*/
  Gain1 : Gain  Gain=1/(2*pi)
  Gain9 : Gain  Gain=mavarage_filter_frequency_base_order
  Zero-Order Hold : ZeroOrderHold  SampleTime=ts_afe
  Out1 : Outport
  wires:
  Constant2/1 -> Divide/1
  Divide/1 -> Zero-Order Hold/1
  In1/1 -> Gain1/1  "Omega_el"
  Gain9/1 -> Divide/2
  Zero-Order Hold/1 -> Out1/1  "period"
  Gain1/1 -> Gain9/1

== system afe_abc_inv_pmsm/afe_abc_inv_psm_mod1/afe_control/voltage_sequence_avg/average_filter_ccaller/Moving Average Filter2/Reset Trigger ==
  Clock : Clock
  Constant1 : Constant  Value=simlength
  Constant3 : Constant  Value=0
  Constant4 : Constant
  Mod : Math  Operator=mod
  Switch : Switch  Criteria=u2 ~= 0  SaturateOnIntegerOverflow=off  InputSameDT=off
  Zero-Order Hold : ZeroOrderHold  SampleTime=ts_afe
  Out1 : Outport
  wires:
  Constant3/1 -> Switch/1
  Zero-Order Hold/1 -> Mod/1
  Constant4/1 -> Switch/3
  Mod/1 -> Switch/2
  Clock/1 -> Zero-Order Hold/1
  Switch/1 -> Out1/1  "Reset"
  Constant1/1 -> Mod/2

== system afe_abc_inv_pmsm/afe_abc_inv_psm_mod1/afe_control/voltage_sequence_avg/average_filter_ccaller/Moving Average Filter3/Enabled Subsystem ==
  In1 : Inport
  Enable : EnablePort
  Constant2 : Constant
  Divide : Product  Inputs=*/
  Gain1 : Gain  Gain=1/(2*pi)
  Gain9 : Gain  Gain=mavarage_filter_frequency_base_order
  Zero-Order Hold : ZeroOrderHold  SampleTime=ts_afe
  Out1 : Outport
  wires:
  Gain1/1 -> Gain9/1
  Zero-Order Hold/1 -> Out1/1  "period"
  Gain9/1 -> Divide/2
  In1/1 -> Gain1/1  "Omega_el"
  Divide/1 -> Zero-Order Hold/1
  Constant2/1 -> Divide/1

== system afe_abc_inv_pmsm/afe_abc_inv_psm_mod1/afe_control/voltage_sequence_avg/average_filter_ccaller/Moving Average Filter3/Reset Trigger ==
  Clock : Clock
  Constant1 : Constant  Value=simlength
  Constant3 : Constant  Value=0
  Constant4 : Constant
  Mod : Math  Operator=mod
  Switch : Switch  Criteria=u2 ~= 0  SaturateOnIntegerOverflow=off  InputSameDT=off
  Zero-Order Hold : ZeroOrderHold  SampleTime=ts_afe
  Out1 : Outport
  wires:
  Constant1/1 -> Mod/2
  Switch/1 -> Out1/1  "Reset"
  Clock/1 -> Zero-Order Hold/1
  Mod/1 -> Switch/2
  Constant4/1 -> Switch/3
  Zero-Order Hold/1 -> Mod/1
  Constant3/1 -> Switch/1

== system afe_abc_inv_pmsm/afe_abc_inv_psm_mod1/afe_control/voltage_sequence_avg/average_filter_ccaller/Moving Average Filter4/Enabled Subsystem ==
  In1 : Inport
  Enable : EnablePort
  Constant2 : Constant
  Divide : Product  Inputs=*/
  Gain1 : Gain  Gain=1/(2*pi)
  Gain9 : Gain  Gain=mavarage_filter_frequency_base_order
  Zero-Order Hold : ZeroOrderHold  SampleTime=ts_afe
  Out1 : Outport
  wires:
  Constant2/1 -> Divide/1
  Divide/1 -> Zero-Order Hold/1
  In1/1 -> Gain1/1  "Omega_el"
  Gain9/1 -> Divide/2
  Zero-Order Hold/1 -> Out1/1  "period"
  Gain1/1 -> Gain9/1

== system afe_abc_inv_pmsm/afe_abc_inv_psm_mod1/afe_control/voltage_sequence_avg/average_filter_ccaller/Moving Average Filter4/Reset Trigger ==
  Clock : Clock
  Constant1 : Constant  Value=simlength
  Constant3 : Constant  Value=0
  Constant4 : Constant
  Mod : Math  Operator=mod
  Switch : Switch  Criteria=u2 ~= 0  SaturateOnIntegerOverflow=off  InputSameDT=off
  Zero-Order Hold : ZeroOrderHold  SampleTime=ts_afe
  Out1 : Outport
  wires:
  Constant3/1 -> Switch/1
  Zero-Order Hold/1 -> Mod/1
  Constant4/1 -> Switch/3
  Mod/1 -> Switch/2
  Clock/1 -> Zero-Order Hold/1
  Switch/1 -> Out1/1  "Reset"
  Constant1/1 -> Mod/2

== system afe_abc_inv_pmsm/afe_abc_inv_psm_mod1/inverter/inverter/sv_pwm/modulator1/PWM generator 1 ==
  m_index : Inport
  phase : Inport  Port=2
  Clock : Clock
  Constant : Constant  Value=dead_time*f
  Constant1 : Constant  Value=polarity
  Constant2 : Constant  Value=1/f
  Constant4 : Constant
  Data Type Conversion1 : DataTypeConversion
  Data Type Conversion2 : DataTypeConversion
  Gain4 : Gain  Gain=1/2
  Gain5 : Gain  Gain=1/(pi/2)
  Hit Crossing : HitCross  ShowOutputPort=off
  Hit Crossing1 : HitCross  ShowOutputPort=off
  MATLAB Function : MATLAB Function  TreatAsAtomicUnit=on
  Relational Operator1 : RelationalOperator  Operator=<=  InputSameDT=off
  Relational Operator2 : RelationalOperator  Operator=<=  InputSameDT=off
  Relay : Relay  OnOutputValue=pos_cmd_gate  OffOutputValue=neg_cmd_gate
  Relay1 : Relay  OnOutputValue=pos_cmd_gate  OffOutputValue=neg_cmd_gate
  Saturation1 : Saturate  UpperLimit=m_up  LowerLimit=m_low
  Sum : Sum  Inputs=|++  SaturateOnIntegerOverflow=on
  Sum1 : Sum  Inputs=-+|  SaturateOnIntegerOverflow=on
  Sum3 : Sum  Inputs=|++
  Switch : Switch  Criteria=u2 > Threshold  SaturateOnIntegerOverflow=off  InputSameDT=off
  Switch1 : Switch  Criteria=u2 > Threshold  SaturateOnIntegerOverflow=off  InputSameDT=off
  m1 : Outport
  m2 : Outport  Port=2
  wires:
  Relational Operator1/1 -> Data Type Conversion1/1
  m_index/1 -> Saturation1/1
  Relational Operator2/1 -> Data Type Conversion2/1
  Data Type Conversion2/1 -> Switch/1, Switch1/3, Hit Crossing1/1
  Constant/1 -> Sum/2, Sum1/1
  Saturation1/1 -> Sum/1, Sum1/2
  Sum/1 -> Relational Operator1/1
  Sum1/1 -> Relational Operator2/2
  Gain4/1 -> Relational Operator2/1, Relational Operator1/2
  Data Type Conversion1/1 -> Hit Crossing/1, Switch/3, Switch1/1
  Switch/1 -> Relay/1
  Clock/1 -> MATLAB Function/1(t)
  Constant2/1 -> MATLAB Function/3(period)
  phase/1 -> MATLAB Function/2(phase)
  MATLAB Function/1(y) -> Gain5/1
  Gain5/1 -> Sum3/1
  Sum3/1 -> Gain4/1
  Constant4/1 -> Sum3/2
  Relay/1 -> m2/1
  Constant1/1 -> Switch1/2, Switch/2
  Switch1/1 -> Relay1/1
  Relay1/1 -> m1/1

== system afe_abc_inv_pmsm/afe_abc_inv_psm_mod1/inverter/inverter/sv_pwm/modulator1/PWM generator 2 ==
  m_index : Inport
  phase : Inport  Port=2
  Clock : Clock
  Constant : Constant  Value=dead_time*f
  Constant1 : Constant  Value=polarity
  Constant2 : Constant  Value=1/f
  Constant4 : Constant
  Data Type Conversion1 : DataTypeConversion
  Data Type Conversion2 : DataTypeConversion
  Gain4 : Gain  Gain=1/2
  Gain5 : Gain  Gain=1/(pi/2)
  Hit Crossing : HitCross  ShowOutputPort=off
  Hit Crossing1 : HitCross  ShowOutputPort=off
  MATLAB Function : MATLAB Function  TreatAsAtomicUnit=on
  Relational Operator1 : RelationalOperator  Operator=<=  InputSameDT=off
  Relational Operator2 : RelationalOperator  Operator=<=  InputSameDT=off
  Relay : Relay  OnOutputValue=pos_cmd_gate  OffOutputValue=neg_cmd_gate
  Relay1 : Relay  OnOutputValue=pos_cmd_gate  OffOutputValue=neg_cmd_gate
  Saturation1 : Saturate  UpperLimit=m_up  LowerLimit=m_low
  Sum : Sum  Inputs=|++  SaturateOnIntegerOverflow=on
  Sum1 : Sum  Inputs=-+|  SaturateOnIntegerOverflow=on
  Sum3 : Sum  Inputs=|++
  Switch : Switch  Criteria=u2 > Threshold  SaturateOnIntegerOverflow=off  InputSameDT=off
  Switch1 : Switch  Criteria=u2 > Threshold  SaturateOnIntegerOverflow=off  InputSameDT=off
  m1 : Outport
  m2 : Outport  Port=2
  wires:
  Relay1/1 -> m1/1
  Switch1/1 -> Relay1/1
  Constant1/1 -> Switch/2, Switch1/2
  Relay/1 -> m2/1
  Constant4/1 -> Sum3/2
  Sum3/1 -> Gain4/1
  Gain5/1 -> Sum3/1
  MATLAB Function/1(y) -> Gain5/1
  phase/1 -> MATLAB Function/2(phase)
  Constant2/1 -> MATLAB Function/3(period)
  Clock/1 -> MATLAB Function/1(t)
  Switch/1 -> Relay/1
  Data Type Conversion1/1 -> Switch1/1, Switch/3, Hit Crossing/1
  Gain4/1 -> Relational Operator1/2, Relational Operator2/1
  Sum1/1 -> Relational Operator2/2
  Sum/1 -> Relational Operator1/1
  Saturation1/1 -> Sum1/2, Sum/1
  Constant/1 -> Sum1/1, Sum/2
  Data Type Conversion2/1 -> Hit Crossing1/1, Switch1/3, Switch/1
  Relational Operator2/1 -> Data Type Conversion2/1
  m_index/1 -> Saturation1/1
  Relational Operator1/1 -> Data Type Conversion1/1

== system afe_abc_inv_pmsm/afe_abc_inv_psm_mod1/inverter/inverter/sv_pwm/modulator1/PWM generator 3 ==
  m_index : Inport
  phase : Inport  Port=2
  Clock : Clock
  Constant : Constant  Value=dead_time*f
  Constant1 : Constant  Value=polarity
  Constant2 : Constant  Value=1/f
  Constant4 : Constant
  Data Type Conversion1 : DataTypeConversion
  Data Type Conversion2 : DataTypeConversion
  Gain4 : Gain  Gain=1/2
  Gain5 : Gain  Gain=1/(pi/2)
  Hit Crossing : HitCross  ShowOutputPort=off
  Hit Crossing1 : HitCross  ShowOutputPort=off
  MATLAB Function : MATLAB Function  TreatAsAtomicUnit=on
  Relational Operator1 : RelationalOperator  Operator=<=  InputSameDT=off
  Relational Operator2 : RelationalOperator  Operator=<=  InputSameDT=off
  Relay : Relay  OnOutputValue=pos_cmd_gate  OffOutputValue=neg_cmd_gate
  Relay1 : Relay  OnOutputValue=pos_cmd_gate  OffOutputValue=neg_cmd_gate
  Saturation1 : Saturate  UpperLimit=m_up  LowerLimit=m_low
  Sum : Sum  Inputs=|++  SaturateOnIntegerOverflow=on
  Sum1 : Sum  Inputs=-+|  SaturateOnIntegerOverflow=on
  Sum3 : Sum  Inputs=|++
  Switch : Switch  Criteria=u2 > Threshold  SaturateOnIntegerOverflow=off  InputSameDT=off
  Switch1 : Switch  Criteria=u2 > Threshold  SaturateOnIntegerOverflow=off  InputSameDT=off
  m1 : Outport
  m2 : Outport  Port=2
  wires:
  Relational Operator1/1 -> Data Type Conversion1/1
  m_index/1 -> Saturation1/1
  Relational Operator2/1 -> Data Type Conversion2/1
  Data Type Conversion2/1 -> Switch/1, Switch1/3, Hit Crossing1/1
  Constant/1 -> Sum/2, Sum1/1
  Saturation1/1 -> Sum/1, Sum1/2
  Sum/1 -> Relational Operator1/1
  Sum1/1 -> Relational Operator2/2
  Gain4/1 -> Relational Operator2/1, Relational Operator1/2
  Data Type Conversion1/1 -> Hit Crossing/1, Switch/3, Switch1/1
  Switch/1 -> Relay/1
  Clock/1 -> MATLAB Function/1(t)
  Constant2/1 -> MATLAB Function/3(period)
  phase/1 -> MATLAB Function/2(phase)
  MATLAB Function/1(y) -> Gain5/1
  Gain5/1 -> Sum3/1
  Sum3/1 -> Gain4/1
  Constant4/1 -> Sum3/2
  Relay/1 -> m2/1
  Constant1/1 -> Switch1/2, Switch/2
  Switch1/1 -> Relay1/1
  Relay1/1 -> m1/1

== system afe_abc_inv_pmsm/afe_abc_inv_psm_mod1/inverter_control/current_ctrl/bemf_observer/bemf_observer/double_integrator_observer ==
  theta : Inport
  Dead Zone : DeadZone  LowerValue=-0.01  UpperValue=0.01
  Gain : Gain  Gain=kw
  Gain1 : Gain  Gain=kg
  Gain2 : Gain  Gain=omega_bez
  Gain3 : Gain  Gain=1/omega_bez
  Gain5 : Gain  Gain=ts_inv
  Sum : Sum  Inputs=-+|
  Sum1 : Sum  Inputs=|++
  Sum2 : Sum  Inputs=|++
  Sum8 : Sum  Inputs=++|
  Unit Delay1 : UnitDelay  InitialCondition=pi  SampleTime=ts_inv  HasFrameUpgradeWarning=on
  Unit Delay2 : UnitDelay  SampleTime=ts_inv  HasFrameUpgradeWarning=on
  bounder1 : MATLAB Function  TreatAsAtomicUnit=on  SystemSampleTime=ts_inv
  bounder2 : MATLAB Function  TreatAsAtomicUnit=on  SystemSampleTime=ts_inv
  omega_pu_hat : Outport  VectorParamsAs1DForOutWhenUnconnected=off
  theta_hat : Outport  Port=2  VectorParamsAs1DForOutWhenUnconnected=off
  wires:
  Gain1/1 -> Sum2/1
  theta/1 -> Sum/2  "theta_bemf"
  Sum8/1 -> Unit Delay1/1
  Unit Delay1/1 -> bounder2/1(u)
  Sum1/1 -> Unit Delay2/1
  Gain/1 -> Gain3/1
  Unit Delay2/1 -> omega_pu_hat/1, Sum1/2, Gain5/1
  Sum2/1 -> Sum8/2
  bounder2/1(y) -> Sum2/2, theta_hat/1, Sum/1  "theta_hat"
  bounder1/1(y) -> Gain1/1, Gain/1
  Gain2/1 -> Sum8/1
  Gain3/1 -> Sum1/1
  Gain5/1 -> Gain2/1
  Sum/1 -> bounder1/1(u)
